simulink model "current_controlled_VSC_ami8p2_simscape"  (R2017b)
settings: Solver=VariableStepAuto  StartTime=0.0  StopTime=0.5  FixedStep=2e-5  MaxStep=2e-5  RelTol=1e-3
InitFcn:
  | current_controlled_VSC_ami8p2_design
values from neighbouring files (symbols this model uses):
  ki = (R+Rz+ron)/taui    [current_controlled_VSC_ami8p2_design.m]
  kp = (L+Lz)/taui    [current_controlled_VSC_ami8p2_design.m]
  L = 100e-6    (= 0.0001)    [current_controlled_VSC_ami8p2_init.m]
  omega0 = 2*pi*60    (= 376.991118431)    [current_controlled_VSC_ami8p2_init.m]
  R = 0.75e-3    (= 0.00075)    [current_controlled_VSC_ami8p2_init.m]
  TimeSample = 1e-6    (= 1e-06)    [current_controlled_VSC_ami8p2_init.m]
  VDC = 1250    [current_controlled_VSC_ami8p2_init.m]
undefined symbols (not defined in the file or in its folder): gcbh, magnitude, pe_sli_rtmsupport, PLL_wmax, PLL_wmin, sigbuilder_block
libraries: nesl_utility x11, pe_lib x9, fl_lib x5, cstblocks x3, powerlib_meascontrol x2, simulink x2, peGeneralControl x1, pePwmGeneratorTwoLevel x1
settings Model: PauseTimes=0.2  Creator=divenyi  LastModifiedBy=divenyi

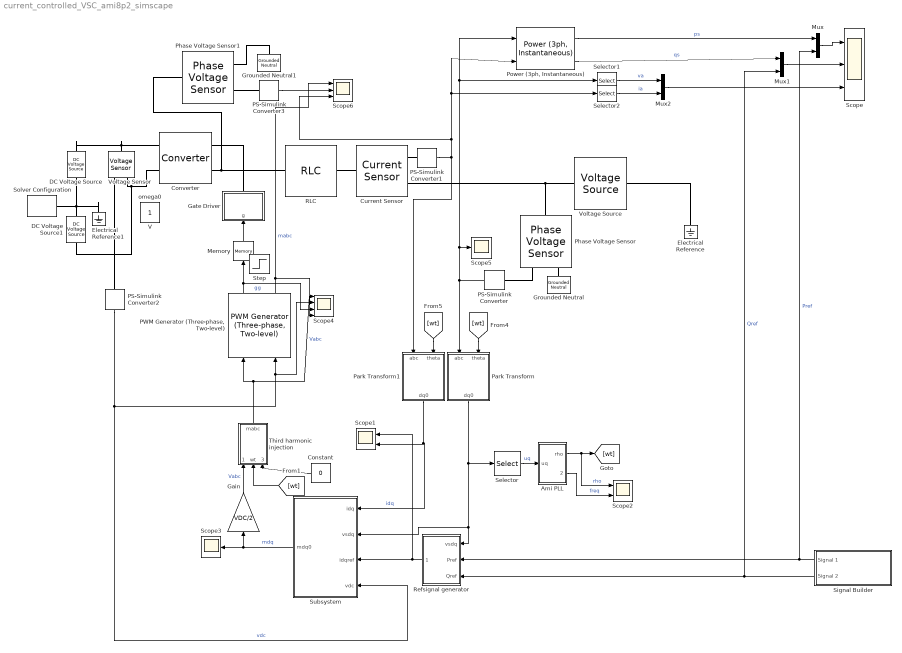
== system current_controlled_VSC_ami8p2_simscape ==
  Ami PLL : Subsystem
  Constant : Constant  Value=0
  Converter : pe_lib/Semiconductors/Converter  device_type=2  Vf=Vd V  Ron=ron Ohm  Rds=0.001 Ohm  Goff=1e-5 1/Ohm  Vth=0.1 V  Vgt=1 V  Vgt_off=-1 V  Ih=1 A  diode_param=2  diode_Vf=Vd V  diode_Ron=0.001 Ohm  diode_Goff=1e-5 1/Ohm  diode_C=50 nF  diode_iRM=-235 A  diode_iF=300 A  diode_idot=-50 A/us  diode_trr_param=1  diode_trr_factor=3  diode_trr=15 us  diode_Qrr=1.5e+3 s*uA  snubber_type=0  Rs=0.1 Ohm  Cs=1e-7 F
      settings: SourceProductName=Simscape Power Systems  SourceProductBaseCode=PS
  Current Sensor : pe_lib/Sensors/Current Sensor
      settings: SourceProductName=Simscape Power Systems  SourceProductBaseCode=PS
  DC Voltage Source : fl_lib/Electrical/Electrical Sources/DC Voltage Source  v0=VDC/2 V
  DC Voltage Source1 : fl_lib/Electrical/Electrical Sources/DC Voltage Source  v0=VDC/2 V
  Electrical Reference : fl_lib/Electrical/Electrical Elements/Electrical Reference
  Electrical Reference1 : fl_lib/Electrical/Electrical Elements/Electrical Reference
  Gain : Gain  Gain=VDC/2
  Gate Driver : Subsystem
  Grounded Neutral : pe_lib/Connections/Grounded Neutral
      settings: SourceProductName=Simscape Power Systems  SourceProductBaseCode=PS
  Grounded Neutral1 : pe_lib/Connections/Grounded Neutral
      settings: SourceProductName=Simscape Power Systems  SourceProductBaseCode=PS
  Memory : Memory
  Mux : Mux  Inputs=2
  Mux1 : Mux  Inputs=2
  Mux2 : Mux  Inputs=2
  PS-Simulink Converter{,1..3} (4 alike) : nesl_utility/PS-Simulink Converter  PhysicalDomain=network_engine_domain  SubClassName=ps_output  LeftPortType=input  RightPortType=output  PseudoPeriodic=off  Frequencies=[]  Unit=1  AffineConversion=off
  "PWM Generator (Three-phase, Two-level)" : pePwmGeneratorTwoLevel/PWM Generator (Three-phase, Two-level)  OverrideUsingVariant=NaturalMode  PWMMode=Continuous PWM (CPWM)  CPWMMode=SPWM: sinusoidal PWM  DPWMMode=60 DPWM: 60 degree discontinuous PWM  fsw=fs  Ts=TimeSample
      settings: SamplingMode=Natural
  Park Transform : Subsystem  AncestorBlock=peTransforms/Park Transform  LoadFcn=pe_sli_rtmsupport( 'loadfcn', gcbh );  mask(Park Transform){AxisAlignment=Q-axis, PowerInvariant=off}
      mask prompts: AxisAlignment "Phase-a axis alignment:"; PowerInvariant "Power invariant"
      mask help: This block implements a rotating reference frame transformation commonly known as the Park transform.
      mask init:
      | if PowerInvariant==0
      |     K1 = 0.5;
      |     K2 = 2/3;
      | else
      |     K1 = 1/sqrt(2);
      |     K2 = sqrt(2/3);
      | end
      | 
      | switch AxisAlignment
      |     case 'Q-axis'
      |         Offset = 0;
      |     case 'D-axis'
      |         Offset = pi/2;
      |     otherwise
      | end
      settings: CopyFcn=pe_sli_rtmsupport( 'copyfcn', gcbh );  DeleteFcn=pe_sli_rtmsupport( 'deletefcn', gcbh );  ModelCloseFcn=pe_sli_rtmsupport( 'modelclosefcn', gcbh );  PostSaveFcn=pe_sli_rtmsupport( 'postsavefcn', gcbh );  PreCopyFcn=pe_sli_rtmsupport( 'precopyfcn', gcbh );  OpenFcn=pe_sli_rtmsupport( 'openfcn', gcbh );  CloseFcn=pe_sli_rtmsupport( 'closefcn', gcbh );  PreDeleteFcn=pe_sli_rtmsupport( 'predeletefcn', gcbh );
      mask Help: web(nesl_help(gcbh))
      mask TypeOptions AxisAlignment: Q-axis | D-axis
      mask Display: pe.mask.drawParkTransform();
  Park Transform1 : Subsystem  AncestorBlock=peTransforms/Park Transform  LoadFcn=pe_sli_rtmsupport( 'loadfcn', gcbh );  mask(Park Transform){AxisAlignment=Q-axis, PowerInvariant=off}
      mask prompts: AxisAlignment "Phase-a axis alignment:"; PowerInvariant "Power invariant"
      mask help: This block implements a rotating reference frame transformation commonly known as the Park transform.
      mask init: same as current_controlled_VSC_ami8p2_simscape/Park Transform
      settings: CopyFcn=pe_sli_rtmsupport( 'copyfcn', gcbh );  DeleteFcn=pe_sli_rtmsupport( 'deletefcn', gcbh );  ModelCloseFcn=pe_sli_rtmsupport( 'modelclosefcn', gcbh );  PostSaveFcn=pe_sli_rtmsupport( 'postsavefcn', gcbh );  PreCopyFcn=pe_sli_rtmsupport( 'precopyfcn', gcbh );  OpenFcn=pe_sli_rtmsupport( 'openfcn', gcbh );  CloseFcn=pe_sli_rtmsupport( 'closefcn', gcbh );  PreDeleteFcn=pe_sli_rtmsupport( 'predeletefcn', gcbh );
      mask Help: web(nesl_help(gcbh))
      mask TypeOptions AxisAlignment: Q-axis | D-axis
      mask Display: pe.mask.drawParkTransform();
  Phase Voltage Sensor : pe_lib/Sensors/Phase Voltage Sensor
      settings: SourceProductName=Simscape Power Systems  SourceProductBaseCode=PS
  Phase Voltage Sensor1 : pe_lib/Sensors/Phase Voltage Sensor
      settings: SourceProductName=Simscape Power Systems  SourceProductBaseCode=PS
  "Power (3ph, Instantaneous)" : powerlib_meascontrol/Measurements/Power (3ph, Instantaneous)
      settings: SourceProductName=Simscape Power Systems
  RLC : pe_lib/Passive Devices/RLC  component_structure=4  R=R Ohm  L=L H  IL0=[0, 0, 0] A  C=1e-6 F  VC0=[0, 0, 0] V  R_parasitic=1e-6 Ohm  G_parasitic=1e-6 1/Ohm
      settings: SourceProductName=Simscape Power Systems  SourceProductBaseCode=PS
  Refsignal generator : Subsystem
  Scope : Scope  NumInputPorts=3
  Scope1 : Scope  NumInputPorts=2
  Scope2 : Scope  NumInputPorts=2
  Scope3 : Scope
  Scope4 : Scope  NumInputPorts=4
  Scope5 : Scope
  Scope6 : Scope  NumInputPorts=3
  Selector : Selector  InputPortWidth=2  IndexOptions=Index vector (dialog)  Indices=[2]  OutputSizes=1
  Selector1 : Selector  InputPortWidth=3  IndexOptions=Index vector (dialog)  Indices=[1]  OutputSizes=1
  Selector2 : Selector  InputPortWidth=3  IndexOptions=Index vector (dialog)  Indices=[1]  OutputSizes=1
  Signal Builder : Subsystem  Tag=STV Subsys  LoadFcn=sigbuilder_block('load');  StartFcn=sigbuilder_block('start');  StopFcn=sigbuilder_block('stop');  ClipboardFcn=sigbuilder_block('clipboard');  mask(Sigbuilder block){tuvar=[0:10]}
      mask help: Simulink:masks:SigbuilderBlock_MD
      mask init:
      | if ~strcmp(get_param(bdroot(gcbh),'SimulationStatus'),'stopped') tuvar = sigbuilder_block('maskInit'); end
      settings: CopyFcn=sigbuilder_block('copy');  DeleteFcn=sigbuilder_block('delete');  ModelCloseFcn=sigbuilder_block('modelClose');  PreSaveFcn=sigbuilder_block('preSave');  PauseFcn=sigbuilder_block('pause');  ContinueFcn=sigbuilder_block('continue');  NameChangeFcn=sigbuilder_block('namechange');  OpenFcn=sigbuilder_block('open',[437.6 199.2 550.4 400 ]);  CloseFcn=sigbuilder_block('close');
      mask Display: plot(0, 0, 100, 100,[2, 2, 32, 32, 2], [68, 8, 8, 68, 68],[32, 2], [38, 38], [32, 19, 2],[53, 60, 44], [32, 17, 17, 2],[16, 16, 31, 31]);txt = getActiveGroup(gcbh);text(2, 100, txt,'verticalAlignment', 'top');
  Solver Configuration : nesl_utility/Solver Configuration  PhysicalDomain=network_engine_domain  SubClassName=solver  LeftPortType=input  RightPortType=generic  Accelerate=off  Tones=[]  Harmonics=[]  SimulateNoise=off  Profile=off  UseLocalSampling=off  EnableSwitchedLinearOptims=on  FrequencyDomain=off  UseCCode=off  RelTol=0.001  AbsTol=1e-06  MinStep=1e-09  ToWorkspace=off  RevertToSquareIcSolve=off  NumHomotopyIterations=100  PhasorMode=off  PhasorModeNumHarmonics=1  DoDC=off  ResidualTolerance=1e-09  UseLocalSolver=off  LocalSolverChoice=NE_BACKWARD_EULER_ADVANCER  LocalSolverSampleTime=TimeSample  DoFixedCost=off  MaxNonlinIter=3  MaxModeIter=2  LinearAlgebra=Sparse  DelaysMemoryBudget=1024  AutomaticFiltering=on  FilteringTimeConstant=0.001
  Subsystem : Subsystem
  "Third harmonic injection " : Subsystem
  Voltage Sensor : fl_lib/Electrical/Electrical Sensors/Voltage Sensor
  Voltage Source : pe_lib/Sources/Voltage Source  vline_rms=Vn V  shift=0 deg  freq=omega0/2/pi Hz  impedance_option=0  SShortCircuit=1e6 V*A  XR=15  R=0.01 Ohm  L=3.97e-4 H  G_parasitic=0 1/Ohm  harmonic_option=0  harmonic_orders=[5, 7, 11, 13]  harmonic_ratios=[.1, .1, .1, .1]  I_specify=off  I_priority=None  I=[ 0 0 0 ] A  I_nominal_specify=off  I_nominal_unit=A  I_nominal_value=1
      settings: SourceProductName=Simscape Power Systems  SourceProductBaseCode=PS
  Step : Step  IOType=siggen  SampleTime=0
  V : Constant  IOType=siggen
  omega0 : Constant  IOType=siggen
  wires:
  Ami PLL/1(rho) -> Scope2/1, [wt]  "rho"
  Signal Builder/1(Signal 1) -> Refsignal generator/2(Pref), Mux/2  "Pref"
  Signal Builder/2(Signal 2) -> Refsignal generator/3(Qref), Mux1/2  "Qref"
  Refsignal generator/1(idqref) -> Subsystem/3(idqref), Scope1/1
  PS-Simulink Converter2/1 -> Scope4/2, "PWM Generator (Three-phase, Two-level)"/2, Subsystem/4(vdc)  "vdc"
  Selector/1 -> Ami PLL/1(uq)  "uq"
  Park Transform1/1(dq0) -> Subsystem/1(idq), Scope1/2  "idq"
  "Power (3ph, Instantaneous)"/1 -> Mux/1  "ps"
  Mux/1 -> Scope/1
  Mux1/1 -> Scope/2
  "Power (3ph, Instantaneous)"/2 -> Mux1/1  "qs"
  Mux2/1 -> Scope/3
  Selector1/1 -> Mux2/1  "va"
  Selector2/1 -> Mux2/2  "ia"
  Ami PLL/2(freq) -> Scope2/2  "freq"
  Subsystem/1(mdq0) -> Scope3/1, Gain/1  "mdq"
  PS-Simulink Converter/1 -> Park Transform/1(abc), Scope5/1, Selector1/1, "Power (3ph, Instantaneous)"/1
  PS-Simulink Converter1/1 -> Park Transform1/1(abc), Scope6/3, Selector2/1, "Power (3ph, Instantaneous)"/2
  [wt] -> Park Transform/2(theta)
  [wt] -> Park Transform1/2(theta)
  Memory/1 -> Gate Driver/1(g)
  "Third harmonic injection "/1(mabc) -> "PWM Generator (Three-phase, Two-level)"/1, Scope4/1  "Vabc"
  "PWM Generator (Three-phase, Two-level)"/1 -> Scope4/3, Memory/1  "gg"
  Park Transform/1(dq0) -> Refsignal generator/1(vsdq), Subsystem/2(vsdq), Selector/1
  "PWM Generator (Three-phase, Two-level)"/2 -> Scope6/1, Scope4/4  "mabc"
  Constant/1 -> "Third harmonic injection "/3(enable)
  Gain/1 -> "Third harmonic injection "/1(mdq)  "Vabc"
  [wt] -> "Third harmonic injection "/2(wt)
  PS-Simulink Converter3/1 -> Scope6/2
  connections:
  Current Sensor/RConn2 -- Phase Voltage Sensor/LConn1 -- Voltage Source/RConn1
  Converter/LConn2 -- Phase Voltage Sensor1/LConn1 -- RLC/LConn1
  Voltage Source/LConn1 -- Electrical Reference/LConn1
  DC Voltage Source/LConn1 -- Converter/RConn1 -- Voltage Sensor/LConn1
  Voltage Sensor/RConn2 -- DC Voltage Source1/RConn1 -- Converter/RConn2
  Gate Driver/RConn1 -- Converter/LConn1
  RLC/RConn1 -- Current Sensor/LConn1
  PS-Simulink Converter/LConn1 -- Phase Voltage Sensor/RConn1
  Current Sensor/RConn1 -- PS-Simulink Converter1/LConn1
  PS-Simulink Converter2/LConn1 -- Voltage Sensor/RConn1
  Phase Voltage Sensor/RConn2 -- Grounded Neutral/LConn1
  Phase Voltage Sensor1/RConn1 -- PS-Simulink Converter3/LConn1
  Phase Voltage Sensor1/RConn2 -- Grounded Neutral1/LConn1
  DC Voltage Source1/LConn1 -- Electrical Reference1/LConn1 -- DC Voltage Source/RConn1 -- Solver Configuration/RConn1

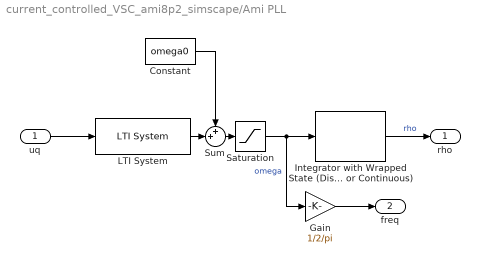
== system current_controlled_VSC_ami8p2_simscape/Ami PLL ==
  uq : Inport
  Constant : Constant  Value=omega0
  Gain : Gain  Gain=1/2/pi
  Integrator with Wrapped State (Discrete or Continuous) : peGeneralControl/Integrator with Wrapped State (Discrete or Continuous)  OverrideUsingVariant=Discrete  WrappedStateUpperValue=2*pi  WrappedStateLowerValue=0  x0=0  Ts=-1
  LTI System : cstblocks/LTI System  sys=PLL_H  IC=[]
  Saturation : Saturate  UpperLimit=PLL_wmax  LowerLimit=PLL_wmin
  Sum : Sum  Inputs=++|
  rho : Outport
  freq : Outport  Port=2
  wires:
  Saturation/1 -> Gain/1, Integrator with Wrapped State (Discrete or Continuous)/1  "omega"
  Integrator with Wrapped State (Discrete or Continuous)/1 -> rho/1  "rho"
  uq/1 -> LTI System/1
  Gain/1 -> freq/1
  LTI System/1 -> Sum/2
  Sum/1 -> Saturation/1
  Constant/1 -> Sum/1

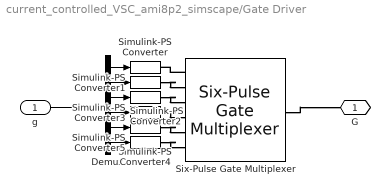
== system current_controlled_VSC_ami8p2_simscape/Gate Driver ==
  g : Inport
  Demux : Demux  Outputs=6
  Simulink-PS Converter{,1..5} (6 alike) : nesl_utility/Simulink-PS Converter  PhysicalDomain=network_engine_domain  SubClassName=ps_input  LeftPortType=input  RightPortType=output  PseudoPeriodic=off  Frequencies=[]  NoiseDistribution=none  NoiseParameters=[]  Unit=1  AffineConversion=off  FilteringAndDerivatives=zero  SimscapeFilterOrder=1  InputFilterTimeConstant=0.001  UdotUserProvided=1
  Six-Pulse Gate Multiplexer : pe_lib/Semiconductors/Six-Pulse Gate Multiplexer  R=0 Ohm
      settings: SourceProductName=Simscape Power Systems  SourceProductBaseCode=PS
  G : PMIOPort  Port=1  Side=Right
  wires:
  Demux/6 -> Simulink-PS Converter5/1
  Demux/5 -> Simulink-PS Converter4/1
  Demux/4 -> Simulink-PS Converter3/1
  Demux/3 -> Simulink-PS Converter2/1
  Demux/2 -> Simulink-PS Converter1/1
  Demux/1 -> Simulink-PS Converter/1
  g/1 -> Demux/1
  connections:
  Six-Pulse Gate Multiplexer/RConn1 -- G/RConn1
  Simulink-PS Converter5/RConn1 -- Six-Pulse Gate Multiplexer/LConn6
  Simulink-PS Converter4/RConn1 -- Six-Pulse Gate Multiplexer/LConn5
  Simulink-PS Converter3/RConn1 -- Six-Pulse Gate Multiplexer/LConn4
  Simulink-PS Converter2/RConn1 -- Six-Pulse Gate Multiplexer/LConn3
  Simulink-PS Converter1/RConn1 -- Six-Pulse Gate Multiplexer/LConn2
  Six-Pulse Gate Multiplexer/LConn1 -- Simulink-PS Converter/RConn1

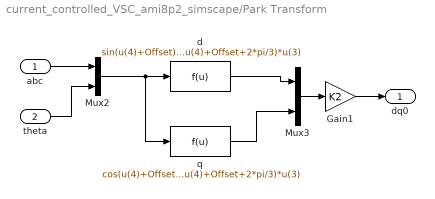
== system current_controlled_VSC_ami8p2_simscape/Park Transform ==
  abc : Inport
  theta : Inport  Port=2
  Gain1 : Gain  Gain=K2
  Mux2 : Mux  Inputs=2
  Mux3 : Mux  Inputs=2
  d : Fcn  Expr=sin(u(4)+Offset)*u(1) + sin(u(4)+Offset-2*pi/3)*u(2) + sin(u(4)+Offset+2*pi/3)*u(3)
  q : Fcn  Expr=cos(u(4)+Offset)*u(1) + cos(u(4)+Offset-2*pi/3)*u(2) + cos(u(4)+Offset+2*pi/3)*u(3)
  dq0 : Outport
  wires:
  abc/1 -> Mux2/1
  d/1 -> Mux3/1
  q/1 -> Mux3/2
  theta/1 -> Mux2/2
  Mux2/1 -> d/1, q/1
  Mux3/1 -> Gain1/1
  Gain1/1 -> dq0/1

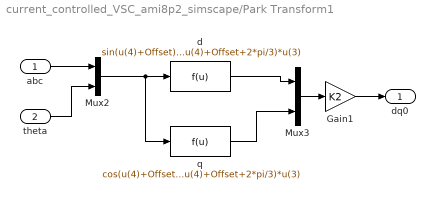
== system current_controlled_VSC_ami8p2_simscape/Park Transform1 ==
  abc : Inport
  theta : Inport  Port=2
  Gain1 : Gain  Gain=K2
  Mux2 : Mux  Inputs=2
  Mux3 : Mux  Inputs=2
  d : Fcn  Expr=sin(u(4)+Offset)*u(1) + sin(u(4)+Offset-2*pi/3)*u(2) + sin(u(4)+Offset+2*pi/3)*u(3)
  q : Fcn  Expr=cos(u(4)+Offset)*u(1) + cos(u(4)+Offset-2*pi/3)*u(2) + cos(u(4)+Offset+2*pi/3)*u(3)
  dq0 : Outport
  wires:
  Gain1/1 -> dq0/1
  Mux3/1 -> Gain1/1
  Mux2/1 -> q/1, d/1
  theta/1 -> Mux2/2
  q/1 -> Mux3/2
  d/1 -> Mux3/1
  abc/1 -> Mux2/1

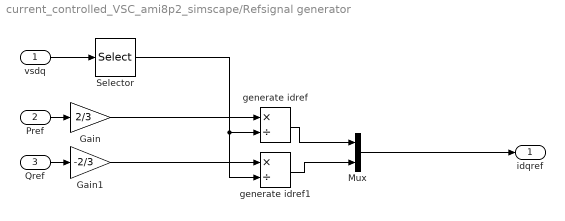
== system current_controlled_VSC_ami8p2_simscape/Refsignal generator ==
  vsdq : Inport
  Pref : Inport  Port=2
  Qref : Inport  Port=3
  Gain : Gain  Gain=2/3
  Gain1 : Gain  Gain=-2/3
  Mux : Mux  Inputs=2
  Selector : Selector  InputPortWidth=2  IndexOptions=Index vector (dialog)  Indices=[1]  OutputSizes=1
  generate idref : Product  Inputs=*/
  generate idref1 : Product  Inputs=*/
  idqref : Outport
  wires:
  Gain/1 -> generate idref/1
  Pref/1 -> Gain/1
  Qref/1 -> Gain1/1
  Gain1/1 -> generate idref1/1
  vsdq/1 -> Selector/1
  generate idref/1 -> Mux/1
  generate idref1/1 -> Mux/2
  Selector/1 -> generate idref/2, generate idref1/2
  Mux/1 -> idqref/1

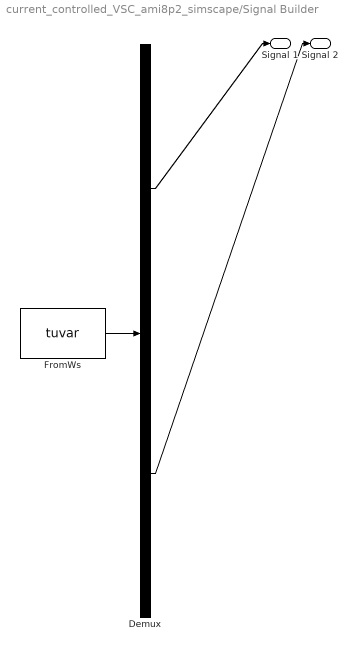
== system current_controlled_VSC_ami8p2_simscape/Signal Builder ==
  Demux : Demux  Tag=STV Demux  Outputs=2
  FromWs : FromWorkspace  Tag=STV FromWs  VariableName=tuvar  SampleTime=0
      SigBuilderData=|
      | common.afterFinalStr = 'Extrapolate'
      | common.sampleTime = 0
      | dataSet.timeRange = [0 0.5]
      | dataSet.name = 'Group 1'
      | sbobj.Groups.Name = 'Group 1'
      | sbobj.Groups.Signals(1).Name = 'Signal 1'
      | sbobj.Groups.Signals(1).XData = [0 0.2 0.2 0.3 0.3 0.5]
      | sbobj.Groups.Signals(1).YData = [0 0 2500000 2500000 -2500000 -2500000]
      | sbobj.Groups.Signals(2).Name = 'Signal 2'
      | sbobj.Groups.Signals(2).XData = [0 0.35 0.35 0.5]
      | sbobj.Groups.Signals(2).YData = [100 100 1000000 1000000]
      | sbobj.Groups.TimeRange = [0 0.5]
  Signal 1 : Outport  Tag=STV Outport
  Signal 2 : Outport  Tag=STV Outport  Port=2
  wires:
  Demux/1 -> Signal 1/1
  FromWs/1 -> Demux/1
  Demux/2 -> Signal 2/1

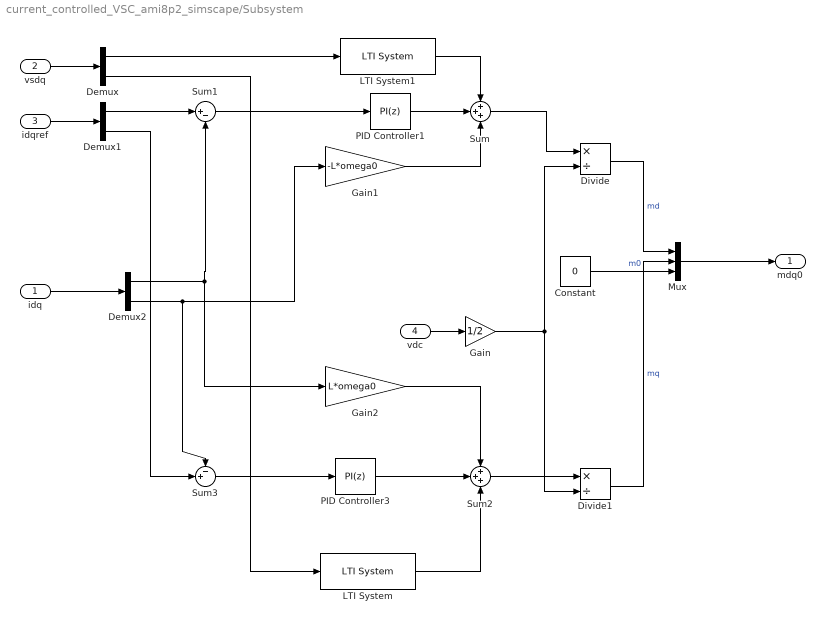
== system current_controlled_VSC_ami8p2_simscape/Subsystem ==
  idq : Inport
  vsdq : Inport  Port=2
  idqref : Inport  Port=3
  vdc : Inport  Port=4
  Constant : Constant  Value=0
  Demux : Demux  Outputs=2
  Demux1 : Demux  Outputs=2
  Demux2 : Demux  Outputs=2
  Divide : Product  Inputs=*/
  Divide1 : Product  Inputs=*/
  Gain : Gain  Gain=1/2
  Gain1 : Gain  Gain=-L*omega0
  Gain2 : Gain  Gain=L*omega0
  LTI System : cstblocks/LTI System  sys=Gff  IC=[]
  LTI System1 : cstblocks/LTI System  sys=Gff  IC=[]
  Mux : Mux  Inputs=3
  PID Controller1 : simulink/Continuous/PID Controller  Controller=PI  TimeDomain=Discrete-time  SampleTime=-1  IntegratorMethod=Forward Euler  FilterMethod=Forward Euler  Form=Parallel  UseFilter=on  ControllerParametersSource=internal  P=kp  I=ki  D=0  N=100  InitialConditionSource=internal  InitialConditionForIntegrator=0  InitialConditionForFilter=0  ExternalReset=none  LimitOutput=off  UpperSaturationLimit=inf  LowerSaturationLimit=-inf  LinearizeAsGain=on  AntiWindupMode=none  Kb=1  TrackingMode=off  Kt=1  PParamMin=[]  PParamMax=[]  IParamMin=[]  IParamMax=[]  DParamMin=[]  DParamMax=[]  NParamMin=[]  NParamMax=[]  KbParamMin=[]  KbParamMax=[]  KtParamMin=[]  KtParamMax=[]  POutMin=[]  POutMax=[]  IOutMin=[]  IOutMax=[]  DOutMin=[]  DOutMax=[]  NOutMin=[]  NOutMax=[]  KbOutMin=[]  KbOutMax=[]  KtOutMin=[]  KtOutMax=[]  IntegratorOutMin=[]  IntegratorOutMax=[]  FilterOutMin=[]  FilterOutMax=[]  SumOutMin=[]  SumOutMax=[]  SumI1OutMin=[]  SumI1OutMax=[]  SumI2OutMin=[]  SumI2OutMax=[]  SumI3OutMin=[]  SumI3OutMax=[]  SumDOutMin=[]  SumDOutMax=[]  SaturationOutMin=[]  SaturationOutMax=[]  IntegratorContinuousStateAttributes=''  IntegratorStateMustResolveToSignalObject=off  IntegratorRTWStateStorageClass=Auto  FilterContinuousStateAttributes=''  FilterStateMustResolveToSignalObject=off  FilterRTWStateStorageClass=Auto  DifferentiatorICPrevScaledInput=0  DifferentiatorOutMin=[]  DifferentiatorOutMax=[]  InitialConditionSetting=State (most efficient)  FilterDiffOutCoefMin=[]  FilterDiffOutCoefMax=[]  SumDenOutMin=[]  SumDenOutMax=[]  SumNumOutMin=[]  SumNumOutMax=[]  ReciprocalOutMin=[]  ReciprocalOutMax=[]  DivideOutMin=[]  DivideOutMax=[]  TunerSelectOption=Transfer Function Based (PID Tuner App)
  PID Controller3 : simulink/Continuous/PID Controller  Controller=PI  TimeDomain=Discrete-time  SampleTime=-1  IntegratorMethod=Forward Euler  FilterMethod=Forward Euler  Form=Parallel  UseFilter=on  ControllerParametersSource=internal  P=kp  I=ki  D=0  N=100  InitialConditionSource=internal  InitialConditionForIntegrator=0  InitialConditionForFilter=0  ExternalReset=none  LimitOutput=off  UpperSaturationLimit=inf  LowerSaturationLimit=-inf  LinearizeAsGain=on  AntiWindupMode=none  Kb=1  TrackingMode=off  Kt=1  PParamMin=[]  PParamMax=[]  IParamMin=[]  IParamMax=[]  DParamMin=[]  DParamMax=[]  NParamMin=[]  NParamMax=[]  KbParamMin=[]  KbParamMax=[]  KtParamMin=[]  KtParamMax=[]  POutMin=[]  POutMax=[]  IOutMin=[]  IOutMax=[]  DOutMin=[]  DOutMax=[]  NOutMin=[]  NOutMax=[]  KbOutMin=[]  KbOutMax=[]  KtOutMin=[]  KtOutMax=[]  IntegratorOutMin=[]  IntegratorOutMax=[]  FilterOutMin=[]  FilterOutMax=[]  SumOutMin=[]  SumOutMax=[]  SumI1OutMin=[]  SumI1OutMax=[]  SumI2OutMin=[]  SumI2OutMax=[]  SumI3OutMin=[]  SumI3OutMax=[]  SumDOutMin=[]  SumDOutMax=[]  SaturationOutMin=[]  SaturationOutMax=[]  IntegratorContinuousStateAttributes=''  IntegratorStateMustResolveToSignalObject=off  IntegratorRTWStateStorageClass=Auto  FilterContinuousStateAttributes=''  FilterStateMustResolveToSignalObject=off  FilterRTWStateStorageClass=Auto  DifferentiatorICPrevScaledInput=0  DifferentiatorOutMin=[]  DifferentiatorOutMax=[]  InitialConditionSetting=State (most efficient)  FilterDiffOutCoefMin=[]  FilterDiffOutCoefMax=[]  SumDenOutMin=[]  SumDenOutMax=[]  SumNumOutMin=[]  SumNumOutMax=[]  ReciprocalOutMin=[]  ReciprocalOutMax=[]  DivideOutMin=[]  DivideOutMax=[]  TunerSelectOption=Transfer Function Based (PID Tuner App)
  Sum : Sum  Inputs=+++
  Sum1 : Sum  Inputs=|+-
  Sum2 : Sum  Inputs=+++
  Sum3 : Sum  Inputs=-+|
  mdq0 : Outport
  wires:
  vdc/1 -> Gain/1
  Gain/1 -> Divide1/2, Divide/2
  Sum/1 -> Divide/1
  Divide/1 -> Mux/1  "md"
  Constant/1 -> Mux/3  "m0"
  Mux/1 -> mdq0/1
  vsdq/1 -> Demux/1
  idqref/1 -> Demux1/1
  Demux1/1 -> Sum1/1
  idq/1 -> Demux2/1
  Gain1/1 -> Sum/3
  Gain2/1 -> Sum2/1
  Demux2/1 -> Gain2/1, Sum1/2
  Demux2/2 -> Gain1/1, Sum3/1
  Demux1/2 -> Sum3/2
  PID Controller3/1 -> Sum2/2
  Sum3/1 -> PID Controller3/1
  Sum2/1 -> Divide1/1
  Divide1/1 -> Mux/2  "mq"
  Demux/2 -> LTI System/1
  Demux/1 -> LTI System1/1
  Sum1/1 -> PID Controller1/1
  PID Controller1/1 -> Sum/2
  LTI System/1 -> Sum2/3
  LTI System1/1 -> Sum/1

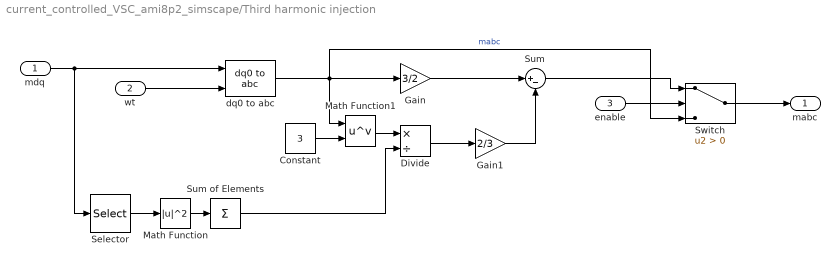
== system current_controlled_VSC_ami8p2_simscape/Third harmonic injection  ==
  mdq : Inport
  wt : Inport  Port=2
  enable : Inport  Port=3
  Constant : Constant  Value=3
  Divide : Product  Inputs=*/
  Gain : Gain  Gain=3/2
  Gain1 : Gain  Gain=2/3
  Math Function : Math  Operator=magnitude^2  SaturateOnIntegerOverflow=on
  Math Function1 : Math  Operator=pow  SaturateOnIntegerOverflow=on
  Selector : Selector  InputPortWidth=3  IndexOptions=Index vector (dialog)  Indices=[1 2]  OutputSizes=1
  Sum : Sum  Inputs=|+-
  Sum of Elements : Sum  Inputs=+
  Switch : Switch  Criteria=u2 > Threshold
  dq0 to abc : powerlib_meascontrol/Transformations/dq0 to abc  Alignment=90 degrees behind phase A axis
  mabc : Outport
  wires:
  Sum/1 -> Switch/1
  enable/1 -> Switch/2
  Switch/1 -> mabc/1
  Gain1/1 -> Sum/2
  Gain/1 -> Sum/1
  Divide/1 -> Gain1/1
  Sum of Elements/1 -> Divide/2
  Math Function1/1 -> Divide/1
  Constant/1 -> Math Function1/2
  Math Function/1 -> Sum of Elements/1
  Selector/1 -> Math Function/1
  mdq/1 -> dq0 to abc/1, Selector/1
  wt/1 -> dq0 to abc/2
  dq0 to abc/1 -> Gain/1, Math Function1/1, Switch/3  "mabc"
